simulink model "JX_Kinect"  (Simulink 7.7)
settings: Solver=ode45  StartTime=0.0  StopTime=inf  FixedStep=sample_time  RelTol=1e-3
InitFcn:
  | sample_time=0.01;
undefined symbols (not defined in the file or in its folder): gray
libraries: vrlib x4, simulink_extras x3, nid_lib x2, vipsnks x1, utility x1
(part 2 of 2)

== matlab function Kinect Roll Pitch Trigger/R Hand Vector ==
  data: x input double; y input double; z input double; y1 output double
function y1 = fcn(x,y,z)
%#codegen
y1 = [x,y,z];

== matlab function Kinect Roll Pitch Trigger/R elbow ==
  data: x input double; y input double; z input double; y1 output double
function y1 = fcn(x,y,z)
%#codegen
y1 = [x,y,z];

== matlab function Kinect Roll Pitch Trigger/R shoulder ==
  data: x input double; y input double; z input double; y1 output double
function y1 = fcn(x,y,z)
%#codegen
y1 = [x,y,z];
